simulink model "model"  (R2024b)
settings: Solver=FixedStepAuto  StartTime=0.0  StopTime=100e-6  RelTol=1e-3
InitFcn:
  | run('../matlab_code/parameters.m')
undefined symbols (not defined in the file): buck_freq, delay
libraries: simulink_extras x2, simulink x2, spsSampleandHoldLib x2, fuzblock x1, spspowerguiLib x1
settings Model: LastModifiedBy=deso
settings OptimizationCC: BlockReduction=off  ConditionallyExecuteInputs=off  OptimizeBlockIOStorage=off  OptimizeDataStoreBuffers=off  BusAssignmentInplaceUpdate=off
settings DebuggingCC: SFUnexpectedBacktrackingDiag=warning  SFNoUnconditionalDefaultTransitionDiag=warning
settings HardwareCC: ProdBitPerPointer=32  ProdBitPerSizeT=32  ProdBitPerPtrDiffT=32  ProdWordSize=32  ProdLongLongMode=on  ProdHWDeviceType=Intel->x86-32 (Windows32)
settings RTWCC: GenCodeOnly=on  GenerateReport=on  BuildConfiguration=Debug  LaunchReport=on
settings CodeAppCC: ForceParamTrailComments=on  MATLABSourceComments=on  EnableCustomComments=on
settings GRTTargetCC: CombineSignalStateStructs=on  SupportVariableSizeSignals=on  MultiInstanceErrorCode=Warning

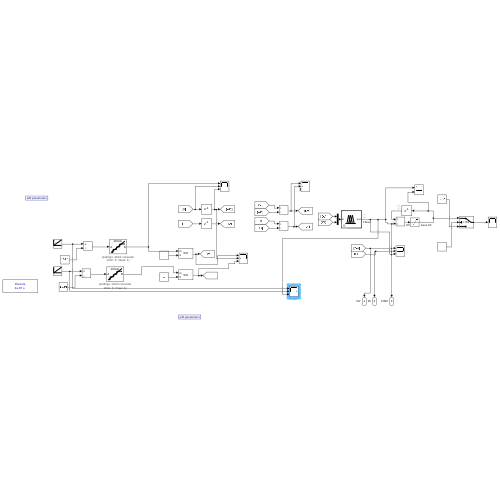
[thumbnail: Simulink's stored preview of the top-level diagram]
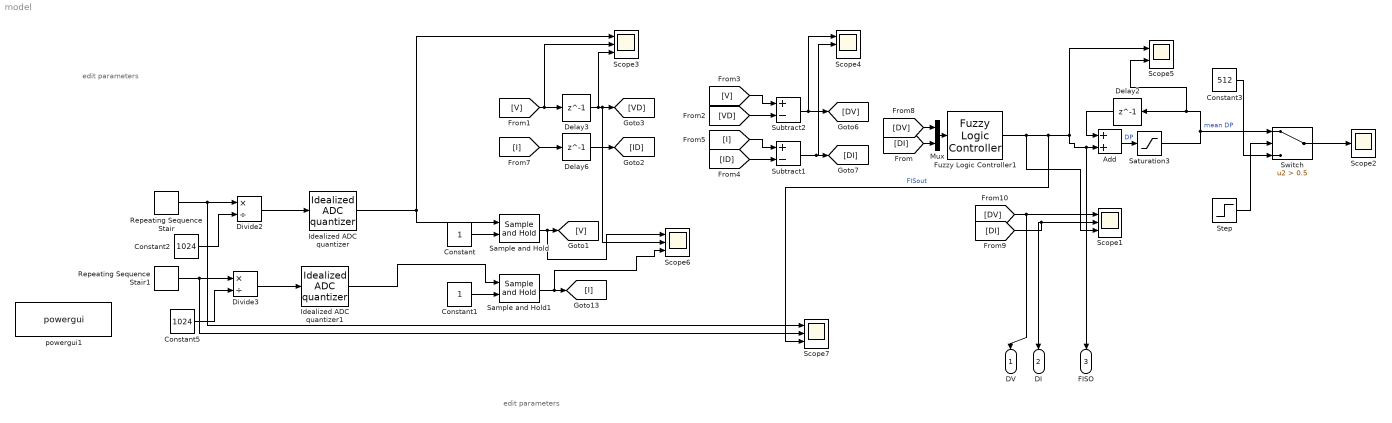
== system model ==
  note: edit parameters
  note: edit parameters
  Add : Sum
  Constant : Constant
  Constant1 : Constant
  Constant2 : Constant  Value=1024
  Constant3 : Constant  Value=512
  Constant5 : Constant  Value=1024
  Delay2 : Delay  DelayLength=1  SampleTime=delay
  Delay3 : Delay  DelayLength=1  SampleTime=delay
  Delay6 : Delay  DelayLength=1  SampleTime=delay
  Divide2 : Product  Inputs=*/
  Divide3 : Product  Inputs=*/
  Fuzzy Logic Controller1 : fuzblock/Fuzzy Logic  Controller  FIS='../FIS_RULES/mpptfuzzy.fis'  OutputSampleNumber=101  DataType=double  FuzzifiedInputs=off  RuleFiringStrengths=off  RuleOutputs=off  AggregatedOutputs=off  SimulateUsing=Interpreted execution  OutOfRangeInputValueMessage=warning  NoRuleFiredMessage=warning  EmptyOutputFuzzySetMessage=warning
  Idealized ADC quantizer : simulink_extras/Additional Discrete/Idealized ADC quantizer  NumberOfConverterBits=10  Vmin=0  Vmax=1  OutputDataType=int16  OutputNegativeValues=off
  Idealized ADC quantizer1 : simulink_extras/Additional Discrete/Idealized ADC quantizer  NumberOfConverterBits=10  Vmin=0  Vmax=1  OutputDataType=int16  OutputNegativeValues=off
  Mux : Mux  Inputs=2
  Repeating Sequence Stair : simulink/Sources/Repeating Sequence Stair  OutValues=[0 10 20 30 40 50 60 70 80 90 100].'  tsamp=delay  OutMin=[]  OutMax=[]  OutDataTypeStr=double  OutputDataTypeScalingMode=double  OutDataType=fixdt(0,8)  ConRadixGroup=Best Precision: Vector-wise  OutScaling=2^-12
  Repeating Sequence Stair1 : simulink/Sources/Repeating Sequence Stair  OutValues=[0 5 10 15 20 25 30 35 40 45 50].'  tsamp=delay  OutMin=[]  OutMax=[]  OutDataTypeStr=double  OutputDataTypeScalingMode=double  OutDataType=fixdt(0,8)  ConRadixGroup=Best Precision: Vector-wise  OutScaling=2^-12
  Sample and Hold : spsSampleandHoldLib/Sample and Hold  ic=0  Ts=delay
      settings: LibrarySourceBlock=|
      | sps_lib/Control/Sample and
      | Hold
  Sample and Hold1 : spsSampleandHoldLib/Sample and Hold  ic=0  Ts=delay
      settings: LibrarySourceBlock=|
      | sps_lib/Control/Sample and
      | Hold
  Saturation3 : Saturate  UpperLimit=716  LowerLimit=307
  Scope{1,3..4,6..7} (5 alike) : Scope  NumInputPorts=3
  Scope2 : Scope
  Scope5 : Scope  NumInputPorts=2
  Step : Step  Time=10e-6  SampleTime=10e-7
  Subtract1 : Sum  Inputs=+-
  Subtract2 : Sum  Inputs=+-
  Switch : Switch  Criteria=u2 > Threshold  Threshold=0.5  SaturateOnIntegerOverflow=off  InputSameDT=off
  powergui1 : spspowerguiLib/powergui  Priority=1  SimulationMode=Discrete  SampleTime=1/(25*buck_freq)  frequency=60  Iterations=50  frequencyindice=0  Pbase=100e6  ErrMax=1e-4  UnitsV=kV  UnitsW=MW  buscounter=0  FunctionMessages=off  echomessages=off  EnableUseOfTLC=off  CurrentSourceSwitches=off  DisableSnubberDevices=off  DisableRonSwitches=off  DisableVfSwitches=off  DisplayEquations=off  AutomaticDiscreteSolvers=off  SolverType=Tustin/Backward Euler (TBE)  Interpol=off  ExternalGateDelay=off  methode=off  Ts=100  x0status=blocks  SPID=on  SwTol=0  HookPort=off  NonlinearTolerance=1e-4  nMaxIteration=100  ContinueOnMaxIteration=off  RestoreLinks=warning  ResistiveCurrentMeasurement=off  Frange=[0:2:500]  Ylog=off  Xlog=on  ShowGrid=off  save=off  variable=ZData  structure=0  ZoomFFT=off  StartTime=0.0  cycles=1  DisplayStyle=1  fundamental=60  FreqAxis=off  MaxFrequency=1000  frequencyindicesteady=1  RmsSteady=1  display=off
  DV : Outport
  DI : Outport  Port=2
  FISO : Outport  Port=3
  wires:
  [VD] -> Subtract2/2
  Repeating Sequence Stair/1 -> Scope7/1, Divide2/1
  Add/1 -> Saturation3/1  "DP"
  [DV] -> Mux/1
  [ID] -> Subtract1/2
  Mux/1 -> Fuzzy Logic Controller1/1
  Idealized ADC quantizer1/1 -> Sample and Hold1/1
  [DI] -> Mux/2
  [I] -> Delay6/1
  [DV] -> DV/1, Scope1/1
  [V] -> Scope3/2, Delay3/1
  Constant1/1 -> Sample and Hold1/2
  Saturation3/1 -> Switch/1, Scope5/2, Delay2/1  "mean DP"
  [DI] -> Scope1/2, DI/1
  Idealized ADC quantizer/1 -> Scope3/1, Sample and Hold/1
  Constant/1 -> Sample and Hold/2
  Delay6/1 -> [ID]
  Fuzzy Logic Controller1/1 -> Scope1/3, Scope7/3, FISO/1, Add/2, Scope5/1  "FISout"
  Subtract1/1 -> Scope4/2, [DI]
  Delay2/1 -> Add/1
  Switch/1 -> Scope2/1
  Divide2/1 -> Idealized ADC quantizer/1
  Delay3/1 -> Scope3/3, Scope6/2, [VD]
  [V] -> Subtract2/1
  Constant3/1 -> Switch/3
  Subtract2/1 -> Scope4/1, [DV]
  Step/1 -> Switch/2
  [I] -> Subtract1/1
  Constant2/1 -> Divide2/2
  Divide3/1 -> Idealized ADC quantizer1/1
  Constant5/1 -> Divide3/2
  Repeating Sequence Stair1/1 -> Scope7/2, Divide3/1
  Sample and Hold/1 -> Scope6/1, [V]
  Sample and Hold1/1 -> Scope6/3, [I]
